simulink model "WECS"  (R2019a)
settings: Solver=FixedStepAuto  StartTime=0.0  StopTime=20  FixedStep=10e-6  RelTol=1e-3
undefined symbols (not defined in the file): DiscIntNeverNeededParam
libraries: powerlib x7, powerlib_meascontrol x3, re_lib x1
settings Model: Creator=BOLT  LastModifiedBy=BOLT

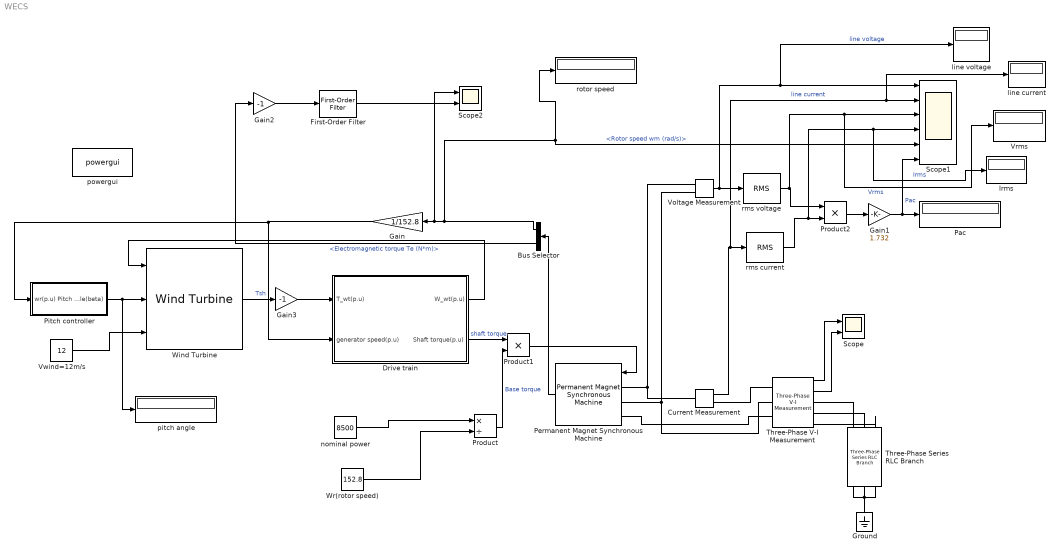
== system WECS ==
  Bus Selector : BusSelector  OutputSignals=Rotor speed wm (rad/s),Electromagnetic torque Te (N*m)
  Current Measurement : powerlib/Measurements/Current Measurement  PhasorSimulation=off  OutputType=Complex  PSBequivalent=0
      settings: SourceProductName=Simscape Electrical
  Drive train : Subsystem
  First-Order Filter : powerlib_meascontrol/Filters/First-Order Filter  FilterType=Lowpass  Tc=1e-3  Ts=50e-6  Initialize=on  Vac_Init=[0, 0, 50]  Vdc_Init=0  PlotResponse=off  FreqRange="[0,  200,  1]"
      settings: SourceProductName=Simscape Electrical
  Gain : Gain  Gain=1/152.8
  Gain1 : Gain  Gain=1.732
  Gain2 : Gain  Gain=-1
  Gain3 : Gain  Gain=-1
  Ground : powerlib/Elements/Ground  LConnTagsString=a
      settings: SourceProductName=Simscape Electrical
  Irms : Display
  Pac : Display
  Permanent Magnet Synchronous Machine : powerlib/Machines/Permanent Magnet Synchronous Machine  NbPhases=3  FluxDistribution=Sinusoidal  RotorType=Round  MechanicalLoad=Torque Tm  PresetModel=No  ShowDetailedParameters=on  MeasurementBus=off  Resistance=0.425  Inductance=8.5e-3  dqInductances=[8.5e-3,8.5e-3]  La=0.000395  MachineConstant=Flux linkage established by magnets (V.s)  Flux=0.433  VoltageCst=392.6876  TorqueCst=3.2475  Flat=120  Mechanical=[0.01197 0.001189 5 0]  PolePairs=4  InitialConditions=[0,0, 0,0]  InitialConditions5ph=[0 0 0 0 0 0]  TsPowergui=0  TsBlock=-1  RefAngle=90 degrees behind phase A axis (modified Park)
  Pitch controller : Subsystem
  Product : Product  Inputs=*/
  Product1 : Product  Inputs=**
  Product2 : Product
  Scope : Scope  NumInputPorts=2
  Scope1 : Scope  NumInputPorts=6
  Scope2 : Scope  NumInputPorts=2
  Three-Phase Series RLC Branch : powerlib/Elements/Three-Phase Series RLC Branch  LConnTagsString=A|B|C  RConnTagsString=A|B|C  BranchType=R  Resistance=25  Inductance=1e-3  Capacitance=1e-6  Measurements=None
      settings: SourceProductName=Simscape Electrical
  Three-Phase V-I Measurement : powerlib/Measurements/Three-Phase V-I Measurement  VoltageMeasurement=phase-to-phase  SetLabelV=off  LabelV=Vabc  Vpu=off  VpuLL=off  CurrentMeasurement=yes  SetLabelI=off  LabelI=Iabc  Ipu=off  Pbase=100e6  Vbase=500e3  OutputType=Complex  PhasorSimulation=off  PSBequivalent=0
      settings: SourceProductName=Simscape Electrical
  Voltage Measurement : powerlib/Measurements/Voltage Measurement  PhasorSimulation=off  OutputType=Complex  PSBequivalent=0
      settings: SourceProductName=Simscape Electrical
  Vrms : Display
  Vwind=12m/s : Constant  Value=12
  Wind Turbine : re_lib/Wind Generation/Wind Turbine  Pnom=8.5e3  Pelec_base=8.5e3/0.9  wind_base=12  P_wind_base=0.8  speed_nom=1  pitch_angle=0  c1_c6="[0.51763          116          0.4            5           21     0.006795]"  cp_nom=0.48  lambda_nom=8.1
      settings: SourceProductName=Simscape Electrical  SourceProductBaseCode=PS
  Wr(rotor speed) : Constant  Value=152.8
  line current : Display
  line voltage : Display
  nominal power : Constant  Value=8500
  pitch angle : Display
  powergui : powerlib/powergui  Priority=1  SimulationMode=Discrete  SampleTime=20e-6  frequency=60  Iterations=50  frequencyindice=0  Pbase=100e6  ErrMax=1e-4  UnitsV=kV  UnitsW=MW  buscounter=0  FunctionMessages=off  echomessages=off  EnableUseOfTLC=off  CurrentSourceSwitches=off  DisableSnubberDevices=off  DisableRonSwitches=off  DisableVfSwitches=off  DisplayEquations=off  AutomaticDiscreteSolvers=off  SolverType=Tustin/Backward Euler (TBE)  Interpol=off  ExternalGateDelay=off  methode=off  Ts=100  x0status=blocks  SPID=on  SwTol=0  HookPort=off  NonlinearTolerance=0  nMaxIteration=15  ContinueOnMaxIteration=off  RestoreLinks=warning  ResistiveCurrentMeasurement=off  Frange=[0:2:500]  Ylog=off  Xlog=on  ShowGrid=off  save=off  variable=ZData  structure=0  ZoomFFT=off  StartTime=0.0  cycles=1  DisplayStyle=1  fundamental=60  FreqAxis=off  MaxFrequency=1000  frequencyindicesteady=1  RmsSteady=1  display=off
      settings: SourceProductName=Simscape Electrical
  rms current : powerlib_meascontrol/Measurements/RMS  TrueRMS=on  Freq=50  RMSInit=120  Ts=50e-6
      settings: SourceProductName=Simscape Electrical
  rms voltage : powerlib_meascontrol/Measurements/RMS  TrueRMS=on  Freq=50  RMSInit=120  Ts=50e-6
      settings: SourceProductName=Simscape Electrical
  rotor speed : Display
  wires:
  Pitch controller/1(Pitch Angle(beta)) -> pitch angle/1, Wind Turbine/2
  Vwind=12m/s/1 -> Wind Turbine/3
  Permanent Magnet Synchronous Machine/1 -> Bus Selector/1
  Bus Selector/1 -> rotor speed/1, Scope1/5, Scope2/1, Gain/1  "<Rotor speed wm (rad/s)>"
  Gain/1 -> Drive train/2(generator speed(p.u)), Pitch controller/1(wr(p.u))
  Drive train/1(W_wt(p.u)) -> Wind Turbine/1
  Drive train/2(Shaft torque(p.u)) -> Product1/1  "shaft torque"
  Product/1 -> Product1/2  "Base torque"
  Wr(rotor speed)/1 -> Product/2
  nominal power/1 -> Product/1
  Product1/1 -> Permanent Magnet Synchronous Machine/1
  Three-Phase V-I Measurement/1 -> Scope/1
  Three-Phase V-I Measurement/2 -> Scope/2
  Voltage Measurement/1 -> line voltage/1, Scope1/1, rms voltage/1  "line voltage"
  Current Measurement/1 -> line current/1, Scope1/2, rms current/1  "line current"
  rms voltage/1 -> Vrms/1, Scope1/3, Product2/1  "Vrms"
  rms current/1 -> Irms/1, Scope1/4, Product2/2  "Irms"
  Product2/1 -> Gain1/1
  Gain1/1 -> Scope1/6, Pac/1  "Pac"
  First-Order Filter/1 -> Scope2/2
  Gain2/1 -> First-Order Filter/1
  Bus Selector/2 -> Gain2/1  "<Electromagnetic torque Te (N*m)>"
  Wind Turbine/1 -> Gain3/1  "Tsh"
  Gain3/1 -> Drive train/1(T_wt(p.u))
  connections:
  Voltage Measurement/LConn1 -- Current Measurement/LConn1 -- Permanent Magnet Synchronous Machine/LConn1
  Three-Phase V-I Measurement/LConn2 -- Voltage Measurement/LConn2 -- Permanent Magnet Synchronous Machine/LConn2
  Three-Phase V-I Measurement/LConn3 -- Permanent Magnet Synchronous Machine/LConn3
  Three-Phase Series RLC Branch/RConn1 -- Ground/LConn1 -- Three-Phase Series RLC Branch/RConn3 -- Three-Phase Series RLC Branch/RConn2
  Three-Phase Series RLC Branch/LConn1 -- Three-Phase V-I Measurement/RConn1
  Three-Phase Series RLC Branch/LConn2 -- Three-Phase V-I Measurement/RConn2
  Three-Phase Series RLC Branch/LConn3 -- Three-Phase V-I Measurement/RConn3
  Three-Phase V-I Measurement/LConn1 -- Current Measurement/RConn1

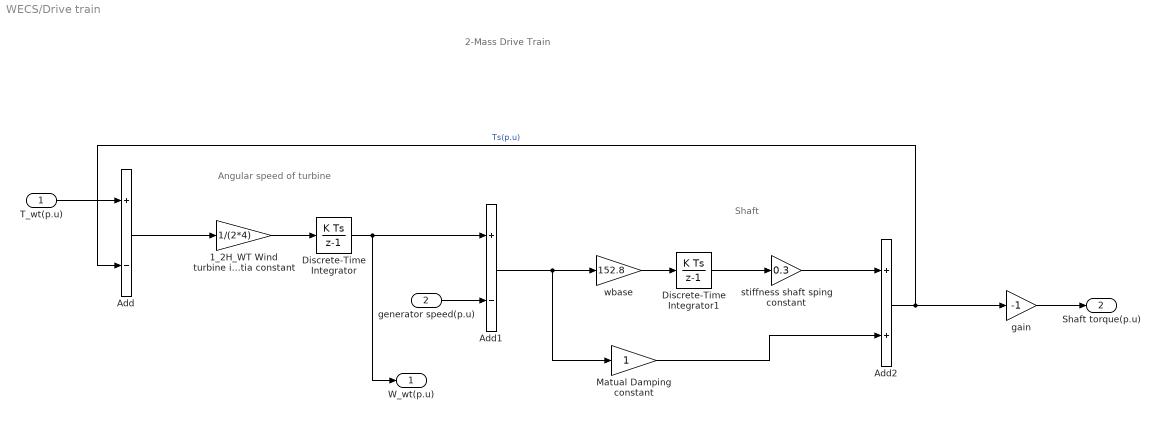
== system WECS/Drive train ==
  note: Shaft
  note: 2-Mass Drive Train
  note: Angular speed of turbine
  T_wt(p.u) : Inport
  generator speed(p.u) : Inport  Port=2
  1_2H_WT Wind turbine inertia constant : Gain  Gain=1/(2*4)
  Add : Sum  Inputs=+-
  Add1 : Sum  Inputs=+-
  Add2 : Sum
  Discrete-Time Integrator : DiscreteIntegrator  InitialCondition=1  SampleTime=50e-6  ICPrevOutput=DiscIntNeverNeededParam  ICPrevScaledInput=DiscIntNeverNeededParam
  Discrete-Time Integrator1 : DiscreteIntegrator  InitialCondition=1/0.3  SampleTime=50e-6  ICPrevOutput=DiscIntNeverNeededParam  ICPrevScaledInput=DiscIntNeverNeededParam
  Matual Damping constant : Gain
  gain : Gain  Gain=-1
  stiffness shaft sping constant : Gain  Gain=0.3
  wbase : Gain  Gain=152.8
  W_wt(p.u) : Outport
  Shaft torque(p.u) : Outport  Port=2
  wires:
  T_wt(p.u)/1 -> Add/1
  Add/1 -> 1_2H_WT Wind turbine inertia constant/1
  1_2H_WT Wind turbine inertia constant/1 -> Discrete-Time Integrator/1
  Discrete-Time Integrator/1 -> W_wt(p.u)/1, Add1/1
  generator speed(p.u)/1 -> Add1/2
  Add1/1 -> Matual Damping constant/1, wbase/1
  wbase/1 -> Discrete-Time Integrator1/1
  Discrete-Time Integrator1/1 -> stiffness shaft sping constant/1
  stiffness shaft sping constant/1 -> Add2/1
  Matual Damping constant/1 -> Add2/2
  Add2/1 -> gain/1, Add/2  "Ts(p.u)"
  gain/1 -> Shaft torque(p.u)/1

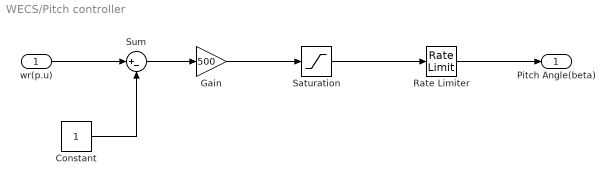
== system WECS/Pitch controller ==
  wr(p.u) : Inport
  Constant : Constant
  Gain : Gain  Gain=500
  Rate Limiter : RateLimiter  RisingSlewLimit=2  FallingSlewLimit=-2  SampleTimeMode=inherited
  Saturation : Saturate  UpperLimit=45  LowerLimit=0
  Sum : Sum  Inputs=|+-
  Pitch Angle(beta) : Outport
  wires:
  wr(p.u)/1 -> Sum/1
  Constant/1 -> Sum/2
  Sum/1 -> Gain/1
  Gain/1 -> Saturation/1
  Saturation/1 -> Rate Limiter/1
  Rate Limiter/1 -> Pitch Angle(beta)/1
